simulink model "Navigation"  (R2025b)
settings: Solver=ode5  StartTime=0.0  StopTime=300  RelTol=1e-3
PostLoadFcn:
  | addpath('settings/')
  | addpath('settings/environment/')
  | 
  | run sensorSettings.m
InitFcn:
  | run main.m
values from neighbouring files (symbols this model uses):
  ba0 = [1;1;1]*0    [main.m]    (also in rocketPlantMain.m = zeros(3,1))
  bg0 = [1;1;1]*0    [main.m]    (also in rocketPlantMain.m = zeros(3,1))
  LLA0 = [deg2rad(lat_deg(1)); deg2rad(lon_deg(1)); 901.0]    [csv_extract.m]    (also in rocketPlantMain.m = [Rocket.Latitude; Rocket.Longitude; Rocket.AltitudeMSL])
  p0 = [0; 0; 0]    [main.m]    (also in rocketPlantMain.m = zeros(3,1))
  P0 = zeros(15, 15)    [main.m]    (also in rocketPlantMain.m = zeros(15,15))
  q0 = q(1,2:5)'    [csv_extract.m]    (also in rocketPlantMain.m = RocketInitialState(7:10))
  stationaryTime = 50    [main.m]    (also in rocketPlantMain.m = Rocket.IgnitionTime)
  v0 = [0;0;0]    [main.m]    (also in rocketPlantMain.m = zeros(3,1))
undefined symbols (not defined in the file or in its folder): DiscIntNeverNeededParam, dspblkCoreblockFVToolHelper, Environment, gcbh, pressure0, Sensor
libraries: simulink x2, dspmathops x1, aerolibutil x1
(part 2 of 3)

== matlab function Navigation/Enviroment/Magnetic Field Model/Magnetic Field Model ==
  data: LLA input; B_ECEF output; g input; h input; Nmax input; t input; alpha_G_0 input; degBool input; B_NED output; B_sph output
function [B_ECEF, B_NED, B_sph] = earthmagfield13(LLA, g, h, Nmax, t, alpha_G_0, degBool)
%
% Earth Magnetic Field with Spherical Harmonics
%
% INPUTS:
%   LLA        [3x1]       [Latitude; Longitude; Altitude]
%                            Latitude  [rad] or [deg]
%                            Longitude [rad] or [deg]
%                            Altitude  [m]
%   g          [14x13]     Gauss coefficient g_nm [T]
%   h          [14x13]     Gauss coefficient h_nm [T]
%   Nmax       [1x1]       Maximum harmonic degree [-]~
%   t          [1x1]       Day Time                       [sec]
%   alpha_G_0  [1x1]       Greenwich Init. Longitude      [rad]
%   degBool    Bool        0 = rad; 1 = deg
%
% OUTPUTS:
%   B_ECEF     [3x1]       Magnetic field in Earth-fixed frame [T]
%   B_NED      [3x1]       Magnetic field in North-East-Down frame [T]
%   B_sph      [3x1]       [B_r; B_theta; B_phi] [T]
%

%% Extract Latitude, Longitude, Altitude from input vector

    lat = LLA(1,1);
    lon = LLA(2,1);
    alt = LLA(3,1) * 1e-3;   % Convert input altitude [m] to [km].

%% Angle handling

    if nargin < 5
        degBool = 0;
    end

    if degBool
        lat = deg2rad(lat);
        lon = deg2rad(lon);
    end

%% Pre-settings

    S_nm   = zeros(Nmax+1, Nmax);
    P_nm   = zeros(Nmax+1, Nmax);
    d_P_nm = zeros(Nmax+1, Nmax);
    K_nm   = zeros(Nmax+1, Nmax);

    g_nm = zeros(Nmax+1, Nmax);
    h_nm = zeros(Nmax+1, Nmax);

    S_00   = 1;
    P_00   = 1;
    d_P_00 = 0;

%% Position from Latitude, Longitude, Altitude

    % Earth reference radius [km]
    Re = 6371;

    % Radius from Earth's center [km]
    r = Re + alt;

    % Latitude
    delta = lat;

    % Co-latitude
    theta = pi/2 - delta;

    % Longitude from Greenwich
    phi = lon;

%% Gauss normalization

    % Coefficients S_n,m
    for j = 1:Nmax
        if j == 1
            S_nm(1,j) = S_00 * ((2*j - 1)/j);
        else
            S_nm(1,j) = S_nm(1,j-1) * ((2*j - 1)/j);
        end
    end

    for j = 1:Nmax
        for i = 2:j+1
            m = i - 1;
            S_nm(i,j) = S_nm(i-1,j) * sqrt( ...
                ((kronDel(1,m) + 1) * (j - m + 1)) / (j + m) );
        end
    end

    % Coefficients K_n,m
    for j = 1:Nmax
        for i = 1:j+1
            m = i - 1;

            if j == 1
                K_nm(i,j) = 0;
            else
                K_nm(i,j) = ((j - 1)^2 - m^2) / ...
                            ((2*j - 1) * (2*j - 3));
            end
        end
    end

%% Associated Legendre functions

    P_nm(1,1) = cos(theta) * P_00;    % P_1,0
    P_nm(2,1) = sin(theta) * P_00;    % P_1,1

    for j = 2:Nmax
        for i = 1:j+1
            m = i - 1;

            if m == j
                P_nm(i,j) = sin(theta) * P_nm(j,j-1);
            else
                if j < 3
                    % Degree zero supplies the missing zonal recurrence term.
                    % For m=1, K_nm is zero at degree two.
                    P_nm(i,j) = cos(theta) * P_nm(i,j-1) ...
                              - K_nm(i,j) * P_00;
                else
                    P_nm(i,j) = cos(theta) * P_nm(i,j-1) ...
                              - K_nm(i,j) * P_nm(i,j-2);
                end
            end
        end
    end

%% Derivatives of associated Legendre functions wrt theta

    d_P_nm(1,1) = cos(theta) * d_P_00 - sin(theta) * P_00;
    d_P_nm(2,1) = sin(theta) * d_P_00 + cos(theta) * P_00;

    for j = 2:Nmax
        for i = 1:j+1
            m = i - 1;

            if m == j
                d_P_nm(i,j) = sin(theta) * d_P_nm(j,j-1) ...
                            + cos(theta) * P_nm(j,j-1);
            else
                if j < 3
                    d_P_nm(i,j) = cos(theta) * d_P_nm(i,j-1) ...
                                - sin(theta) * P_nm(i,j-1) ...
                                - K_nm(i,j) * d_P_00;
                else
                    d_P_nm(i,j) = cos(theta) * d_P_nm(i,j-1) ...
                                - sin(theta) * P_nm(i,j-1) ...
                                - K_nm(i,j) * d_P_nm(i,j-2);
                end
            end
        end
    end

%% Gaussian coefficient normalization

    for j = 1:Nmax
        for i = 1:j+1
            g_nm(i,j) = S_nm(i,j) * g(i,j);
            h_nm(i,j) = S_nm(i,j) * h(i,j);
        end
    end

%% Magnetic field components in spherical coordinates

    % Radial component
    pr = 0;

    for j = 1:Nmax
        dx = 0;
        sx = (Re/r)^(j+2) * (j + 1);

        for i = 1:j+1
            m = i - 1;

            dx = dx + ...
                (g_nm(i,j) * cos(m*phi) + h_nm(i,j) * sin(m*phi)) ...
                * P_nm(i,j);
        end

        pr = pr + sx * dx;
    end

    B_r = pr;

    % Co-latitude component
    pr = 0;

    for j = 1:Nmax
        dx = 0;
        sx = (Re/r)^(j+2);

        for i = 1:j+1
            m = i - 1;

            dx = dx + ...
                (g_nm(i,j) * cos(m*phi) + h_nm(i,j) * sin(m*phi)) ...
                * d_P_nm(i,j);
        end

        pr = pr + sx * dx;
    end

    B_theta = -pr;

    % Longitude / azimuth component
    pr = 0;

    for j = 1:Nmax
        dx = 0;
        sx = (Re/r)^(j+2);

        for i = 1:j+1
            m = i - 1;

            dx = dx + ...
                m * (-g_nm(i,j) * sin(m*phi) + h_nm(i,j) * cos(m*phi)) ...
                * P_nm(i,j);
        end

        pr = pr + sx * dx;
    end

    if abs(sin(theta)) < 1e-12
        B_phi = 0;
    else
        B_phi = -pr / sin(theta);
    end

    B_sph = [B_r; B_theta; B_phi];

%% Convert to local North-East-Down frame

    % e_theta points south, so north = -B_theta
    % e_phi points east
    % radial points upward, so down = -B_r

    B_NED = [-B_theta;
              B_phi;
             -B_r];

%% Convert to Earth-fixed Cartesian frame

    B_1 = (B_r*cos(delta) + B_theta*sin(delta)) * cos(phi) ...
          - B_phi*sin(phi);

    B_2 = (B_r*cos(delta) + B_theta*sin(delta)) * sin(phi) ...
          + B_phi*cos(phi);

    B_3 = B_r*sin(delta) - B_theta*cos(delta);

    B_ECEF = [B_1; B_2; B_3];

end

%% Helper function

function d = kronDel(j,k)
    if j == k
        d = 1;
    else
        d = 0;
    end
end

== matlab function Navigation/Enviroment/NED to LLA ==
  data: p_N input; LLA output; LLA0 input
function LLA = NED2LLA(p_N, LLA0)

    % p_N = [local north; local east; absolute altitude] in meters
    % LLA0 = [lat0; lon0; h0]
    % lat0, lon0 in rad
    % h0 in m
    %
    % LLA output = [lat; lon; h]
    % lat, lon in rad
    % h in m
    
    % WGS-84 constants
    a = 6378137.0;
    e2 = 6.69437999014e-3;
    
    lat0 = LLA0(1);
    lon0 = LLA0(2);
    h0   = LLA0(3);
    
    north = p_N(1);
    east  = p_N(2);
    h = p_N(3);   % Absolute trajectory altitude; do not add h0 again.
    
    sinLat = sin(lat0);
    
    RN = a / sqrt(1 - e2*sinLat^2);
    RM = a*(1 - e2) / (1 - e2*sinLat^2)^(3/2);
    
    lat = lat0 + north/(RM + h0);
    lon = lon0 + east/((RN + h0)*cos(lat0));
    
    LLA = [lat; lon; h];

end

== matlab function Navigation/Magnetic Field Model/Magnetic Field Model ==
  data: LLA input; B_ECEF output; g input; h input; Nmax input; degBool input; B_NED output; B_sph output
function [B_ECEF, B_NED, B_sph] = earthmagfield13(LLA, g, h, Nmax, degBool)
%
% Earth Magnetic Field with Spherical Harmonics
%
% INPUTS:
%   LLA        [3x1]       [Latitude; Longitude; Altitude]
%                            Latitude  [rad] or [deg]
%                            Longitude [rad] or [deg]
%                            Altitude  [m]
%   g          [14x13]     Gauss coefficient g_nm [T]
%   h          [14x13]     Gauss coefficient h_nm [T]
%   Nmax       [1x1]       Maximum harmonic degree [-]
%   degBool    Bool        0 = rad; 1 = deg
%
% OUTPUTS:
%   B_ECEF     [3x1]       Magnetic field in Earth-fixed frame [T]
%   B_NED      [3x1]       Magnetic field in North-East-Down frame [T]
%   B_sph      [3x1]       [B_r; B_theta; B_phi] [T]
%

%% Extract Latitude, Longitude, Altitude from input vector

    lat = LLA(1,1);
    lon = LLA(2,1);
    alt = LLA(3,1) * 1e-3;   % Convert input altitude [m] to [km].

%% Angle handling

    if nargin < 5
        degBool = 0;
    end

    if degBool
        lat = deg2rad(lat);
        lon = deg2rad(lon);
    end

%% Pre-settings

    S_nm   = zeros(Nmax+1, Nmax);
    P_nm   = zeros(Nmax+1, Nmax);
    d_P_nm = zeros(Nmax+1, Nmax);
    K_nm   = zeros(Nmax+1, Nmax);

    g_nm = zeros(Nmax+1, Nmax);
    h_nm = zeros(Nmax+1, Nmax);

    S_00   = 1;
    P_00   = 1;
    d_P_00 = 0;

%% Position from Latitude, Longitude, Altitude

    % Earth reference radius [km]
    Re = 6371;

    % Radius from Earth's center [km]
    r = Re + alt;

    % Latitude
    delta = lat;

    % Co-latitude
    theta = pi/2 - delta;

    % Longitude from Greenwich
    phi = lon;

%% Gauss normalization

    % Coefficients S_n,m
    for j = 1:Nmax
        if j == 1
            S_nm(1,j) = S_00 * ((2*j - 1)/j);
        else
            S_nm(1,j) = S_nm(1,j-1) * ((2*j - 1)/j);
        end
    end

    for j = 1:Nmax
        for i = 2:j+1
            m = i - 1;
            S_nm(i,j) = S_nm(i-1,j) * sqrt( ...
                ((kronDel(1,m) + 1) * (j - m + 1)) / (j + m) );
        end
    end

    % Coefficients K_n,m
    for j = 1:Nmax
        for i = 1:j+1
            m = i - 1;

            if j == 1
                K_nm(i,j) = 0;
            else
                K_nm(i,j) = ((j - 1)^2 - m^2) / ...
                            ((2*j - 1) * (2*j - 3));
            end
        end
    end

%% Associated Legendre functions

    P_nm(1,1) = cos(theta) * P_00;    % P_1,0
    P_nm(2,1) = sin(theta) * P_00;    % P_1,1

    for j = 2:Nmax
        for i = 1:j+1
            m = i - 1;

            if m == j
                P_nm(i,j) = sin(theta) * P_nm(j,j-1);
            else
                if j < 3
                    P_nm(i,j) = cos(theta) * P_nm(i,j-1) ...
                          - K_nm(i,j) * P_00;
                else
                    P_nm(i,j) = cos(theta) * P_nm(i,j-1) ...
                              - K_nm(i,j) * P_nm(i,j-2);
                end
            end
        end
    end

%% Derivatives of associated Legendre functions wrt theta

    d_P_nm(1,1) = cos(theta) * d_P_00 - sin(theta) * P_00;
    d_P_nm(2,1) = sin(theta) * d_P_00 + cos(theta) * P_00;

    for j = 2:Nmax
        for i = 1:j+1
            m = i - 1;

            if m == j
                d_P_nm(i,j) = sin(theta) * d_P_nm(j,j-1) ...
                            + cos(theta) * P_nm(j,j-1);
            else
                if j < 3
                    d_P_nm(i,j) = cos(theta) * d_P_nm(i,j-1) ...
                                - sin(theta) * P_nm(i,j-1) ...
                                - K_nm(i,j) * d_P_00;
                else
                    d_P_nm(i,j) = cos(theta) * d_P_nm(i,j-1) ...
                                - sin(theta) * P_nm(i,j-1) ...
                                - K_nm(i,j) * d_P_nm(i,j-2);
                end
            end
        end
    end

%% Gaussian coefficient normalization

    for j = 1:Nmax
        for i = 1:j+1
            g_nm(i,j) = S_nm(i,j) * g(i,j);
            h_nm(i,j) = S_nm(i,j) * h(i,j);
        end
    end

%% Magnetic field components in spherical coordinates

    % Radial component
    pr = 0;

    for j = 1:Nmax
        dx = 0;
        sx = (Re/r)^(j+2) * (j + 1);

        for i = 1:j+1
            m = i - 1;

            dx = dx + ...
                (g_nm(i,j) * cos(m*phi) + h_nm(i,j) * sin(m*phi)) ...
                * P_nm(i,j);
        end

        pr = pr + sx * dx;
    end

    B_r = pr;

    % Co-latitude component
    pr = 0;

    for j = 1:Nmax
        dx = 0;
        sx = (Re/r)^(j+2);

        for i = 1:j+1
            m = i - 1;

            dx = dx + ...
                (g_nm(i,j) * cos(m*phi) + h_nm(i,j) * sin(m*phi)) ...
                * d_P_nm(i,j);
        end

        pr = pr + sx * dx;
    end

    B_theta = -pr;

    % Longitude / azimuth component
    pr = 0;

    for j = 1:Nmax
        dx = 0;
        sx = (Re/r)^(j+2);

        for i = 1:j+1
            m = i - 1;

            dx = dx + ...
                m * (-g_nm(i,j) * sin(m*phi) + h_nm(i,j) * cos(m*phi)) ...
                * P_nm(i,j);
        end

        pr = pr + sx * dx;
    end

    if abs(sin(theta)) < 1e-12
        B_phi = 0;
    else
        B_phi = -pr / sin(theta);
    end

    B_sph = [B_r; B_theta; B_phi];

%% Convert to local North-East-Down frame

    % e_theta points south, so north = -B_theta
    % e_phi points east
    % radial points upward, so down = -B_r

    B_NED = [-B_theta;
              B_phi;
             -B_r];

%% Convert to Earth-fixed Cartesian frame

    B_1 = (B_r*cos(delta) + B_theta*sin(delta)) * cos(phi) ...
          - B_phi*sin(phi);

    B_2 = (B_r*cos(delta) + B_theta*sin(delta)) * sin(phi) ...
          + B_phi*cos(phi);

    B_3 = B_r*sin(delta) - B_theta*cos(delta);

    B_ECEF = [B_1; B_2; B_3];

end

%% Helper function

function d = kronDel(j,k)
    if j == k
        d = 1;
    else
        d = 0;
    end
end

== matlab function Navigation/Enviroment/System/MATLAB Function1 ==
  data: Cd input; Thrust input; env input; xNext output; t input; xDot output; x input; rocket input; dt input; yNav output; dbg output
function [xNext, xDot, yNav, dbg] = rocketPyEOMv1Nav(Cd, Thrust, env, t, x, rocket, dt)

    % RocketPy EOM v1 inspired MATLAB Function for Simulink.
    %
    % State:
    %   x = [r_I;
    %        v_I;
    %        q_BI;
    %        omega_B]
    %
    % where:
    %   r_I      = [x;y;z] inertial/local position, z up [m]
    %   v_I      = inertial/local velocity [m/s]
    %   q_BI     = [q0;q1;q2;q3], scalar-first quaternion
    %              maps BODY frame to INERTIAL frame
    %   omega_B  = body angular velocity [rad/s]
    %
    % RocketPy convention:
    %   Body axis 3, i.e. body z, is the rocket longitudinal/symmetry axis.
    %   Thrust_B = [0; 0; Thrust].
    %
    % Inputs:
    %   Cd       = drag coefficient [-]
    %   Thrust   = net thrust [N], already pressure-corrected if desired
    %   env      = environment struct/bus
    %   t        = current time [s], kept for Simulink/RocketPy compatibility
    %   x        = 13x1 last state
    %   rocket   = rocket struct/bus with mass, geometry and inertia data
    %   dt       = propagation step [s]
    %
    % Outputs:
    %   xNext    = discrete propagated state
    %   xDot     = continuous derivative
    %   yNav     = ideal navigation outputs
    %   dbg      = debug vector
    %
    % -------------------------------------------------------------------------
    % Required env fields:
    %
    %   env.rho             air density [kg/m^3]
    %   env.wind_I          inertial wind vector [m/s], 3x1
    %   env.speedOfSound    speed of sound [m/s]
    %   env.g               gravity [m/s^2]
    %   env.earthRate_I     Earth rotation vector in local inertial frame [rad/s]
    %                       use [0;0;0] if neglected
    %
    % Required rocket fields:
    %
    %   rocket.area              reference area [m^2]
    %   rocket.refLength         reference length [m]
    %
    %   rocket.mass              current total mass [kg]
    %   rocket.massDot           current dm/dt [kg/s]
    %                            negative during burn if mass decreases
    %   rocket.massDdot          current d2m/dt2 [kg/s^2]
    %
    %   rocket.rCM_B             CM relative to CDM in body frame [m], 3x1
    %   rocket.rCMdot_B          time derivative of rCM_B [m/s], 3x1
    %   rocket.rCMddot_B         second derivative of rCM_B [m/s^2], 3x1
    %
    %   rocket.rNozzle_B         nozzle position relative to CDM [m], 3x1
    %   rocket.Snozzle_B         nozzle gyration tensor, 3x3
    %                            use zeros(3,3) if neglected
    %
    %   rocket.I_B               inertia tensor about CDM in body frame [kg m^2]
    %   rocket.Idot_B            derivative of inertia tensor [kg m^2/s]
    %
    %   rocket.aeroForceExtra_B  extra aero force [N], 3x1
    %                            use [0;0;0] if only axial drag is used
    %   rocket.aeroMomentExtra_B extra aero moment [N m], 3x1
    %                            use [0;0;0] if neglected
    %
    %   rocket.cpEcc_B           CP eccentricity vector [m], 3x1
    %                            usually [cp_ecc_x; cp_ecc_y; 0]
    %   rocket.thrustEcc_B       thrust eccentricity vector [m], 3x1
    %                            usually [thrust_ecc_x; thrust_ecc_y; 0]
    %
    %   rocket.rIMU_B            IMU position relative to CDM [m], 3x1
    %
    % Notes:
    %   - For continuous Simulink integration, use xDot and set dt = 0.
    %   - For discrete propagation, use xNext.
    %   - Cd and Thrust can come from lookup tables generated from RocketPy.
    
    unused_t = t; %#ok<NASGU>
    
    % Normalize quaternion before derivative
    x(7:10) = normalizeQuat(x(7:10));
    
    % Continuous derivative at current state
    [xDot, yNav, dbg] = localDerivative(Cd, Thrust, env, x, rocket);
    
    % Optional RK4 propagation
    if dt > 0
        k1 = xDot;
        k2 = localDerivative(Cd, Thrust, env, x + 0.5*dt*k1, rocket);
        k3 = localDerivative(Cd, Thrust, env, x + 0.5*dt*k2, rocket);
        k4 = localDerivative(Cd, Thrust, env, x + dt*k3, rocket);
    
        xNext = x + dt/6.0*(k1 + 2*k2 + 2*k3 + k4);
        xNext(7:10) = normalizeQuat(xNext(7:10));
    else
        xNext = x;
    end

end

% ======================================================================= %
%                          Equation of Motion                             %
% ======================================================================= %

function [xDot, yNav, dbg] = localDerivative(Cd, Thrust, env, x, rocket)

    % ---------------------------------------------------------------------- %
    % State unpacking
    % ---------------------------------------------------------------------- %
    
    r_I     = x(1:3);
    v_I     = x(4:6);
    q_BI    = normalizeQuat(x(7:10));
    omega_B = x(11:13);
    
    K_BI = quatToDcm(q_BI);   % body -> inertial
    K_IB = K_BI.';            % inertial -> body
    
    % ---------------------------------------------------------------------- %
    % Mass and geometry
    % ---------------------------------------------------------------------- %
    
    m     = max(rocket.mass, 1e-9);
    mDot  = rocket.massDot;
    mDdot = rocket.massDdot;
    
    rCM_B     = rocket.rCM_B;
    rCMdot_B  = rocket.rCMdot_B;
    rCMddot_B = rocket.rCMddot_B;
    rNoz_B    = rocket.rNozzle_B;
    
    I_CDM_B = rocket.I_B;
    Idot_B  = rocket.Idot_B;
    
    Snoz_B = rocket.Snozzle_B;
    
    % RocketPy computes inertia about CM from inertia about CDM
    S_rCM = skew3(rCM_B);
    H = m * (S_rCM * (-S_rCM));
    I_CM_B = I_CDM_B - H;
    
    % Numerical regularization
    I_CM_B = I_CM_B + 1e-9*eye(3);
    
    % ---------------------------------------------------------------------- %
    % Atmosphere and freestream
    % ---------------------------------------------------------------------- %
    
    wind_I = env.wind_I;
    
    % RocketPy freestream convention: free_stream_velocity = wind - velocity
    freeStream_I = wind_I - v_I;
    freeStream_B = K_IB * freeStream_I;
    
    Vinf = norm(freeStream_I);
    Vsafe = max(Vinf, 1e-6);
    
    Mach = Vinf / max(env.speedOfSound, 1e-6);
    qbar = 0.5 * env.rho * Vinf^2;
    
    % RocketPy drag is axial in body axis 3
    R3_drag = -qbar * rocket.area * Cd;
    
    % Extra aero force can include fins, airbrakes, lift, etc.
    R_B = [0; 0; R3_drag] + rocket.aeroForceExtra_B;
    
    % Aerodynamic-stream convention used for alpha/beta diagnostics
    aeroStream_B = -freeStream_B;
    
    alpha = atan2(aeroStream_B(2), max(abs(aeroStream_B(3)), 1e-9));
    beta  = atan2(aeroStream_B(1), max(abs(aeroStream_B(3)), 1e-9));
    
    % ---------------------------------------------------------------------- %
    % Moments
    % ---------------------------------------------------------------------- %
    
    Fthrust_B = [0; 0; Thrust];
    
    % Extra aero moment can include surfaces, damping, roll moment, etc.
    M_B = rocket.aeroMomentExtra_B;
    
    % Eccentricity moments, same structure as RocketPy:
    %   M_cp     = cp_ecc x aero_force
    %   M_thrust = thrust_ecc x thrust_force
    M_B = M_B ...
        + cross(rocket.cpEcc_B, R_B) ...
        + cross(rocket.thrustEcc_B, Fthrust_B);
    
    % ---------------------------------------------------------------------- %
    % Weight in body frame
    % ---------------------------------------------------------------------- %
    
    weight_I = [0; 0; -m * env.g];
    weight_B = K_IB * weight_I;
    
    % ---------------------------------------------------------------------- %
    % RocketPy intermediate terms
    % ---------------------------------------------------------------------- %
    
    T00 = m * rCM_B;
    
    T03 = 2*mDot*(rNoz_B - rCM_B) ...
        - 2*m*rCMdot_B;
    
    T04 = Fthrust_B ...
        - m*rCMddot_B ...
        - 2*mDot*rCMdot_B ...
        + mDdot*(rNoz_B - rCM_B);
    
    T05 = mDot*Snoz_B - Idot_B;
    
    % RocketPy T20:
    %   ((omega x T00) x omega) + omega x T03 + T04 + weight + aero
    T20 = cross(cross(omega_B, T00), omega_B) ...
        + cross(omega_B, T03) ...
        + T04 ...
        + weight_B ...
        + R_B;
    
    % RocketPy T21:
    %   (I omega) x omega + T05 omega - weight x rCM + moments
    T21 = cross(I_CDM_B*omega_B, omega_B) ...
        + T05*omega_B ...
        - cross(weight_B, rCM_B) ...
        + M_B;
    
    % ---------------------------------------------------------------------- %
    % Coupled angular and translational acceleration
    % ---------------------------------------------------------------------- %
    
    omegaDot_B = I_CM_B \ (T21 + cross(T20, rCM_B));
    
    vDot_body_equiv = T20/m - cross(rCM_B, omegaDot_B);
    
    % Transform acceleration to inertial frame and include Earth rotation term
    vDot_I = K_BI * vDot_body_equiv ...
           - 2*cross(env.earthRate_I, v_I);
    
    % ---------------------------------------------------------------------- %
    % Quaternion derivative
    % ---------------------------------------------------------------------- %
    
    qDot = 0.5 * quatOmegaBody(q_BI) * omega_B;
    
    % ---------------------------------------------------------------------- %
    % State derivative
    % ---------------------------------------------------------------------- %
    
    xDot = zeros(13,1);
    xDot(1:3)   = v_I;
    xDot(4:6)   = vDot_I;
    xDot(7:10)  = qDot;
    xDot(11:13) = omegaDot_B;
    
    % ---------------------------------------------------------------------- %
    % Ideal navigation outputs
    % ---------------------------------------------------------------------- %
    
    % IMU acceleration including lever arm
    rIMU_B = rocket.rIMU_B;
    
    aIMU_I = vDot_I ...
           + K_BI*(cross(omegaDot_B, rIMU_B) ...
           + cross(omega_B, cross(omega_B, rIMU_B)));
    
    % Ideal accelerometer specific force
    g_I = [0; 0; -env.g];
    fIMU_B = K_IB * (aIMU_I - g_I);
    
    % yNav layout:
    %   1:3    position inertial [m]
    %   4:6    velocity inertial [m/s]
    %   7:10   quaternion scalar-first [-]
    %   11:13  gyro ideal, omega_B [rad/s]
    %   14:16  accelerometer ideal, specific force body [m/s^2]
    %   17:19  inertial acceleration of CDM [m/s^2]
    %   20     Mach number [-]
    yNav = zeros(20,1);
    yNav(1:3)   = r_I;
    yNav(4:6)   = v_I;
    yNav(7:10)  = q_BI;
    yNav(11:13) = omega_B;
    yNav(14:16) = fIMU_B;
    yNav(17:19) = vDot_I;
    yNav(20)    = Mach;
    
    % dbg layout:
    %   1   Mach
    %   2   dynamic pressure [Pa]
    %   3   freestream speed [m/s]
    %   4   mass [kg]
    %   5   massDot [kg/s]
    %   6   rCM z [m]
    %   7   axial drag R3 [N]
    %   8   norm aero force [N]
    %   9   norm moment [N m]
    %   10  norm omegaDot [rad/s^2]
    %   11  alpha [rad]
    %   12  beta [rad]
    %   13  thrust [N]
    %   14  altitude z [m]
    %   15  norm freeStream_B [m/s]
    %   16  norm fIMU_B [m/s^2]
    dbg = zeros(16,1);
    dbg(1)  = Mach;
    dbg(2)  = qbar;
    dbg(3)  = Vinf;
    dbg(4)  = m;
    dbg(5)  = mDot;
    dbg(6)  = rCM_B(3);
    dbg(7)  = R3_drag;
    dbg(8)  = norm(R_B);
    dbg(9)  = norm(M_B);
    dbg(10) = norm(omegaDot_B);
    dbg(11) = alpha;
    dbg(12) = beta;
    dbg(13) = Thrust;
    dbg(14) = r_I(3);
    dbg(15) = norm(freeStream_B);
    dbg(16) = norm(fIMU_B);

end

% ======================================================================= %
%                              Helpers                                    %
% ======================================================================= %

function q = normalizeQuat(q)

    nq = sqrt(q(1)^2 + q(2)^2 + q(3)^2 + q(4)^2);
    
    if nq < 1e-12
        q = [1; 0; 0; 0];
    else
        q = q / nq;
    end
    
    % Avoid quaternion sign jumps in logs
    if q(1) < 0
        q = -q;
    end

end

function K = quatToDcm(q)

    % Scalar-first quaternion.
    % K maps body frame to inertial frame:
    %   v_I = K * v_B
    
    q = normalizeQuat(q);
    
    q0 = q(1);
    q1 = q(2);
    q2 = q(3);
    q3 = q(4);
    
    K = zeros(3,3);
    
    K(1,1) = 1 - 2*(q2^2 + q3^2);
    K(1,2) = 2*(q1*q2 - q0*q3);
    K(1,3) = 2*(q1*q3 + q0*q2);
    
    K(2,1) = 2*(q1*q2 + q0*q3);
    K(2,2) = 1 - 2*(q1^2 + q3^2);
    K(2,3) = 2*(q2*q3 - q0*q1);
    
    K(3,1) = 2*(q1*q3 - q0*q2);
    K(3,2) = 2*(q2*q3 + q0*q1);
    K(3,3) = 1 - 2*(q1^2 + q2^2);

end

function Q = quatOmegaBody(q)

    q0 = q(1);
    q1 = q(2);
    q2 = q(3);
    q3 = q(4);
    
    Q = [ -q1, -q2, -q3;
           q0, -q3,  q2;
           q3,  q0, -q1;
          -q2,  q1,  q0 ];

end

function S = skew3(v)

    S = [   0, -v(3),  v(2);
          v(3),    0, -v(1);
         -v(2), v(1),    0 ];

end

== matlab function Navigation/ISA Pressure to Altitude3 ==
  data: p input; h output
function h = ISA_pressure_to_altitude(p)

    % ISA pressure-to-altitude conversion for the troposphere.
    %
    % Input:
    %   p : static pressure [Pa]
    %
    % Output:
    %   h : altitude above sea level [m]
    %
    % Assumptions:
    %   - ISA troposphere model
    %   - sea-level pressure p0 = 101325 Pa
    %   - valid approximately for h < 11 km
    
    T0 = 288.15;       % sea-level standard temperature [K]
    L  = 0.0065;       % temperature lapse rate [K/m]
    R  = 287.05;       % specific gas constant for air [J/(kg K)]
    g0 = 9.80665;      % gravitational acceleration [m/s^2]
    p0 = 101325.0;     % sea-level standard pressure [Pa]
    
    exponent = (R * L) / g0;
    
    h = (T0 / L) * (1.0 - (p / p0)^exponent);

end

== matlab function Navigation/Enviroment/System/MATLAB Function2 ==
  data: h input; p output
function p = ISA_altitude_to_pressure(h)

    % ISA altitude-to-pressure conversion for the troposphere.
    %
    % Input:
    %   h : altitude above sea level [m]
    %
    % Output:
    %   p : static pressure [Pa]
    %
    % Assumptions:
    %   - ISA troposphere model
    %   - sea-level pressure p0 = 101325 Pa
    %   - valid approximately for h < 11 km
    
    T0 = 288.15;       % sea-level standard temperature [K]
    L  = 0.0065;       % temperature lapse rate [K/m]
    R  = 287.05;       % specific gas constant for air [J/(kg K)]
    g0 = 9.80665;      % gravitational acceleration [m/s^2]
    p0 = 101325.0;     % sea-level standard pressure [Pa]
    
    exponent = g0 / (R * L);
    
    p = p0 * (1.0 - (L * h) / T0)^exponent;

end

== matlab function Navigation/Enviroment/Gravity Model/MATLAB Function1 ==
  data: h input; lat input; g_n output
function g_n = WGS84_Model(h, lat)
% WGS-84 normal gravity approximation in NED frame.
%
% Inputs:
%   lat   geodetic latitude [rad]
%   h     altitude above ellipsoid [m]
%
% Output:
%   g_n   gravity vector in NED frame [m/s^2]

    Re = 6378137.0;              % WGS-84 semi-major axis [m]
    f  = 1 / 298.257223563;      % flattening
    e2 = f * (2 - f);            % eccentricity squared

    ge = 9.7803253359;           % gravity at equator [m/s^2]
    k  = 0.00193185265241;

    s = sin(lat);

    g0 = ge * (1 + k*s^2) / sqrt(1 - e2*s^2);

    % Altitude correction
    g = g0 * (1 - 2*h/Re + 3*(h/Re)^2);

    % NED: Down is positive
    g_n = [0; 0; g];
end

== matlab function Navigation/Enviroment/System/RRC3 ==
  data: p_Pa input; h_m output
function h_m = RRC3_pressure_to_altitude_m(p_Pa)
% RRC3_pressure_to_altitude_m
% Pressure altitude conversion consistent with the RRC3/NOAA formula.
%
% Input:
%   p_Pa : static pressure [Pa]
%
% Output:
%   h_m : pressure altitude [m]

    h_ft = RRC3_pressure_to_altitude_ft(p_Pa);

    h_m = h_ft .* 0.3048;

end

function h_ft = RRC3_pressure_to_altitude_ft(p_Pa)
% RRC3_pressure_to_altitude_ft
% Pressure altitude conversion consistent with the RRC3/NOAA formula.
%
% Input:
%   p_Pa : static pressure [Pa]
%
% Output:
%   h_ft : pressure altitude [ft]

    p_hPa = p_Pa ./ 100.0;

    h_ft = (1.0 - (p_hPa ./ 1013.25).^0.190284) .* 145366.45;

end

== matlab function Navigation/Enviroment/System/ISA Pressure to Altitude3 ==
  data: p input; h output
function h = ISA_pressure_to_altitude(p)

    % ISA pressure-to-altitude conversion for the troposphere.
    %
    % Input:
    %   p : static pressure [Pa]
    %
    % Output:
    %   h : altitude above sea level [m]
    %
    % Assumptions:
    %   - ISA troposphere model
    %   - sea-level pressure p0 = 101325 Pa
    %   - valid approximately for h < 11 km
    
    T0 = 288.15;       % sea-level standard temperature [K]
    L  = 0.0065;       % temperature lapse rate [K/m]
    R  = 287.05;       % specific gas constant for air [J/(kg K)]
    g0 = 9.80665;      % gravitational acceleration [m/s^2]
    p0 = 101325.0;     % sea-level standard pressure [Pa]
    
    exponent = (R * L) / g0;
    
    h = (T0 / L) * (1.0 - (p / p0)^exponent);

end

== matlab function Navigation/Enviroment/Gravity Model/MATLAB Function ==
  data: g output; h input
function g = gravity_height(h)

    g0 = 9.80665;      % [m/s^2]
    Re = 6371000.0;    % [m]

    g = [0; 0 ;g0 * (Re / (Re + h))^2];

end

== matlab function Navigation/Enviroment/Magnetic Field Model/MATLAB Function1 ==
  data: r_N input; B_N output; t input; g input; h input; alpha_G_0 input; n input
function B_N   = earthmagfield13(r_N, t, g, h, alpha_G_0, n)
%
% Earth Magnetic Field with Spherical Harmonics
%
%DESCRIPTION:
%This code computes the components of the Earth's Magnetic Field using
%spherical harmonics from order 1 until order 13.
%
%--------------------------------------------------------------------------
% INPUTS:
%   r_N        [3x1]       S/C Position in Inertial Frame [km]
%   t          [1x1]       Day Time                       [sec]
%   g          [14x13]     Gauss Coff. g_nm Matrix        [T]
%   h          [14x13]     Gauss Coff. h_nm Matrix        [T]
%   alpha_G_0  [1x1]       Greenwich Init. Longitude      [rad]
%   n          [1x1]       Order Desired                  [-]
%--------------------------------------------------------------------------
% OUTPUTS:
%   B_N        [3x1]       Mag. Field Components     [T]
%--------------------------------------------------------------------------
%% Pre-Settings & Memory Allocation
    %Matrix of Coefficients S_n,m
    S_nm = zeros(n+1,n);
    S_00 = 1;
    %Matrix of Coefficients P^n,m
    P_nm = zeros(n+1,n);
    P_00 = 1;
    %Matrix of Coefficients Derivatives d_P^n,m
    d_P_nm = zeros(n+1,n);
    d_P_00 = 0;
    %Matrix of Coefficients K^n,m
    K_nm = zeros(n+1,n);
    %Matrix of Coefficients g_nm, h_nm
    g_nm = zeros(n+1,n);
    h_nm = zeros(n+1,n);
%% Topocentric Horizon Angles
    z = r_N(3,1);
    x = r_N(1,1);
    y = r_N(2,1);
    ab = norm(r_N);
    %Earth Radius [km]
    Re = 6371;
    %Earth Angular Velocity [rad/sec]
    om_E = 7.292124*1e-5;
    %Elevation (or Declination) = Latitude (no J2 effect)
    delta = asin(z/ab);
    %Coelevation
    theta = pi/2 - delta;
    %Greenwich Meridian Longitude
    alpha_G = alpha_G_0 + t * om_E;
    %Right Ascension (Local Sidereal Time)
    if (y/ab) > 0
        alpha = acos((x/ab)/cos(delta));
    else
        alpha = 2*pi - acos((x/ab)/cos(delta));
    end
    %Longitude (from Greenwich)
    phi = alpha - alpha_G;
%% Gauss Normalization
    %Coefficients S_nm
    %OBS i = m and j = n
    %First Row (S_n,0)
    for j = 1 : n
        if j == 1
            S_nm(1,j) = S_00 * ((2*j - 1)/j);
        elseif j >= 2
            S_nm(1,j) = S_nm(1,j-1)*((2*j - 1)/j);
        end
    end
    %Remaining Components (S_n,m)
    for j = 1 : n
        for i = 2 : j+1
                S_nm(i,j) = S_nm(i-1,j)*sqrt(((kronDel(1,i-1) + 1)*(j - (i-1) + 1))...
                                        /(j + (i -1)));
        end
    end
    %Coefficients K^n,m
    for j = 1 : n
        for i = 1 : j+1
            if j == 1
                K_nm(i,j) = 0;
            elseif j > 1
                K_nm(i,j) = ((j - 1)^2 - (i-1)^2) / ((2*j - 1)*(2*j - 3));
            end
        end
    end
    %Coefficients P^n,m
    P_nm(1,1) = cos(theta)*P_00;        %P_1,0
    P_nm(2,1) = sin(theta)*P_00;        %P_1,1
    for j = 2 : n
        for i = 1 : j+1
            if i-1 == j                             %P_n,n
                P_nm(i,j) = sin(theta)*P_nm(j,j-1);
            else
                if j < 3                            %P_n,m
                    P_nm(i,j) = cos(theta)*P_nm(i,j-1);
                else
                    P_nm(i,j) = cos(theta)*P_nm(i,j-1) - K_nm(i,j)*P_nm(i,j-2);
                end
            end
        end
    end
    %Derivative of d_P^n,m (wrt theta)
    d_P_nm(1,1) = cos(theta)*d_P_00 - sin(theta)*P_00; %d_P_1,0
    d_P_nm(2,1) = sin(theta)*d_P_00 + cos(theta)*P_00; %d_P_1,1
    for j = 2 : n
        for i = 1 : j+1
            if i-1 == j
                d_P_nm(i,j) = sin(theta)*d_P_nm(j,j-1) + cos(theta)*P_nm(j,j-1);
            else
                if j < 3
                    d_P_nm(i,j) = cos(theta)*d_P_nm(i,j-1) - sin(theta)*P_nm(i,j-1);
                else
                    d_P_nm(i,j) = cos(theta)*d_P_nm(i,j-1) - ...
                            sin(theta)*P_nm(i,j-1) - K_nm(i,j)*d_P_nm(i,j-2);
                end
            end
        end
    end
%% Guassian Coefficients Normalization
    for j = 1 : n
        for i = 1 : j+1
            g_nm(i,j) = S_nm(i,j)*g(i,j);
            h_nm(i,j) = S_nm(i,j)*h(i,j);
        end
    end
%% Magnetic Field Components - Spherical Coordinates
    %Reset Handle Variables
    dx = 0;
    pr = 0;
    %Radial Component
    for j = 1 : n
        sx = (Re/norm(r_N))^(j+2) * (j + 1);
        for i = 1 : j+1
            dx = dx + (g_nm(i,j)*cos((i-1)*phi) + h_nm(i,j)*sin((i-1)*phi)) * P_nm(i,j);
        end
        pr = pr + sx*dx;
        dx = 0;
    end
    B_r = pr;
    %Reset Handle Variables
    dx = 0;
    pr = 0;
    %Coelevation Component
    for j = 1 : n
        sx = ((Re/norm(r_N))^(j+2));
        for i = 1 : j+1
            dx = dx + (g_nm(i,j)*cos((i-1)*phi) + h_nm(i,j)*sin((i-1)*phi)) * d_P_nm(i,j);
        end
        pr = pr + sx*dx;
        dx = 0;
    end
    B_th = -pr;
    %Reset Handle Variables
    dx = 0;
    pr = 0;
    %Azimuth Component
    for j = 1 : n
        sx = ((Re/norm(r_N))^(j+2));
        for i = 1 : j+1
            dx = dx + (i*(-g_nm(i,j)*sin((i-1)*phi) + h_nm(i,j)*cos((i-1)*phi)) * P_nm(i,j));
        end
        pr = pr + sx*dx;
        dx = 0;
    end
    B_phi = -1/sin(theta) * pr;
%% Magnetic Field Components - Inertial Ref. Frame
    B_1 = (B_r*cos(delta) + B_th*sin(delta))*cos(alpha) - B_phi*sin(alpha);
    B_2 = (B_r*cos(delta) + B_th*sin(delta))*sin(alpha) + B_phi*cos(alpha);
    B_3 = (B_r*sin(delta) - B_th*cos(delta));
    B_N = [B_1; B_2; B_3];
end

%% Helper Function

function d = kronDel(j,k)
    if j == k
        d = 1;
    else
        d = 0;
    end
end
